simulink model "Md32StEnCtrl"  (R2018b)
settings: Solver=FixedStepDiscrete  StartTime=0.0  StopTime=10.0  FixedStep=0.01  RelTol=1e-3
undefined symbols (not defined in the file or in its folder): data, SecRwLtStBkReclnEn_Clear, SecRwLtStBkReclnEn_Set, SecRwRtStBkReclnEn_Clear, SecRwRtStBkReclnEn_Set, ThdRwLtStBkReclnEn_Clear, ThdRwLtStBkReclnEn_Set, ThdRwLtStCshnFldEn_Clear, ThdRwLtStCshnFldEn_Set
libraries: simulink x1
settings Model: Creator=sn2xws  LastModifiedBy=sn2xws
settings Model: ModifiedHistory=|
  | 2024.6.24 V3.0.0 557模式流程V1.9
  | 2024.8.16 V3.0.1函数增加FirstTrig
  | 2024.8.20 V3.0.2FirstTrig 折叠刀位置时，不再调用电机
  | 2024.12.17 V3.0.3 BUG 962485 3L靠背和2L靠背应同时进行
settings DataIOCC: SaveFormat=StructureWithTime
settings OptimizationCC: DefaultParameterBehavior=Inlined  EnhancedBackFolding=on  PassReuseOutputArgsAs=Individual arguments  ZeroExternalMemoryAtStartup=off  ZeroInternalMemoryAtStartup=off  OptimizeBlockOrder=speed  DifferentSizesBufferReuse=on  OptimizationCustomize=off
settings DebuggingCC: ParameterTunabilityLossMsg=error
settings SFSimCC: MATLABDynamicMemAlloc=off
settings RTWCC: SystemTargetFile=autosar.tlc  GenCodeOnly=on  TemplateMakefile=ert_default_tmf  Description=AUTOSAR  GenerateReport=on  IncludeHyperlinkInReport=on  LaunchReport=on  GenerateTraceInfo=on  GenerateTraceReport=on  GenerateTraceReportSl=on  GenerateTraceReportSf=on  GenerateTraceReportEml=on
settings CodeAppCC: ForceParamTrailComments=on  IgnoreCustomStorageClasses=off  OperatorAnnotations=on  SimulinkDataObjDesc=on  SFDataObjDesc=on  InsertBlockDesc=on
settings STFCustomTargetCC: TargetLangStandard=C99 (ISO)  MultiwordLength=256  ParMdlRefBuildCompliant=on  CompOptLevelCompliant=on  IncludeMdlTerminateFcn=off  CombineOutputUpdateFcns=on  SuppressErrorStatus=on  ERTCustomFileBanners=on  SupportNonFinite=off  SupportComplex=off  SupportContinuousTime=off  SupportNonInlinedSFcns=off  RemoveResetFunc=on  MATLABClassNameForMDSCustomization=Simulink.SoftwareTarget.ERTCustomization  AutosarCompliant=on  UseToolchainInfoCompliant=on  LookupTableObjectStructAxisOrder=2,1,3,4,...  LUTObjectStructOrderEvenSpacing=Size,Table,Breakpoints  SystemTargetFile=autosar.tlc
settings ERTTargetCC: TargetLangStandard=C99 (ISO)  ConcurrentExecutionCompliant=off  IncludeMdlTerminateFcn=off  SuppressErrorStatus=on  SupportNonFinite=off  SupportComplex=off  ModelStepFunctionPrototypeControlCompliant=off  CPPClassGenCompliant=off  AutosarCompliant=on  LookupTableObjectStructAxisOrder=2,1,3,4,...  LUTObjectStructOrderEvenSpacing=Size,Table,Breakpoints  InlinedParameterPlacement=NonHierarchical  ERTCustomFileTemplate=example_file_process.tlc  ERTFilePackagingFormat=Compact

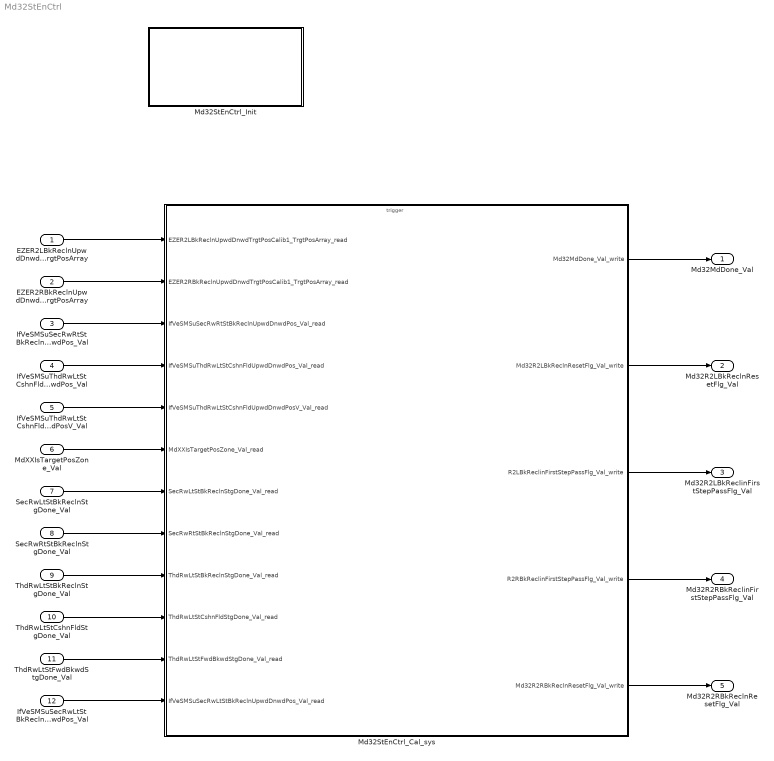
== system Md32StEnCtrl ==
  EZER2LBkReclnUpwdDnwdTrgtPosCalib1_TrgtPosArray : Inport  Description=|  OutDataTypeStr=uint16  PortDimensions=3
      | 0:Pos
      | 1:Max
      | 2:Min
  EZER2RBkReclnUpwdDnwdTrgtPosCalib1_TrgtPosArray : Inport  Description=|  Port=2  OutDataTypeStr=uint16  PortDimensions=3
      | 0:Pos
      | 1:Max
      | 2:Min
  IfVeSMSuSecRwRtStBkReclnUpwdDnwdPos_Val : Inport  Port=3  OutDataTypeStr=uint16  PortDimensions=1
  IfVeSMSuThdRwLtStCshnFldUpwdDnwdPos_Val : Inport  Port=4  OutDataTypeStr=uint16  PortDimensions=1
  IfVeSMSuThdRwLtStCshnFldUpwdDnwdPosV_Val : Inport  Port=5  OutDataTypeStr=boolean  PortDimensions=1
  MdXXIsTargetPosZone_Val : Inport  Port=6  OutDataTypeStr=uint32  PortDimensions=1
  SecRwLtStBkReclnStgDone_Val : Inport  Port=7  OutDataTypeStr=boolean  PortDimensions=1
  SecRwRtStBkReclnStgDone_Val : Inport  Port=8  OutDataTypeStr=boolean  PortDimensions=1
  ThdRwLtStBkReclnStgDone_Val : Inport  Port=9  OutDataTypeStr=boolean  PortDimensions=1
  ThdRwLtStCshnFldStgDone_Val : Inport  Port=10  OutDataTypeStr=boolean  PortDimensions=1
  ThdRwLtStFwdBkwdStgDone_Val : Inport  Port=11  OutDataTypeStr=boolean  PortDimensions=1
  IfVeSMSuSecRwLtStBkReclnUpwdDnwdPos_Val : Inport  Port=12  OutDataTypeStr=uint16  PortDimensions=1
  Md32StEnCtrl_Cal_sys : Subsystem
  Md32StEnCtrl_Init : Subsystem
  Md32MdDone_Val : Outport  OutDataTypeStr=uint8  PortDimensions=1
  Md32R2LBkReclnResetFlg_Val : Outport  Port=2  OutDataTypeStr=boolean  PortDimensions=1
  Md32R2LBkReclinFirstStepPassFlg_Val : Outport  Port=3  OutDataTypeStr=boolean  PortDimensions=1
  Md32R2RBkReclinFirstStepPassFlg_Val : Outport  Port=4  OutDataTypeStr=boolean  PortDimensions=1
  Md32R2RBkReclnResetFlg_Val : Outport  Port=5  OutDataTypeStr=boolean  PortDimensions=1
  wires:
  EZER2LBkReclnUpwdDnwdTrgtPosCalib1_TrgtPosArray/1 -> Md32StEnCtrl_Cal_sys/1(EZER2LBkReclnUpwdDnwdTrgtPosCalib1_TrgtPosArray_read)
  EZER2RBkReclnUpwdDnwdTrgtPosCalib1_TrgtPosArray/1 -> Md32StEnCtrl_Cal_sys/2(EZER2RBkReclnUpwdDnwdTrgtPosCalib1_TrgtPosArray_read)
  IfVeSMSuSecRwRtStBkReclnUpwdDnwdPos_Val/1 -> Md32StEnCtrl_Cal_sys/3(IfVeSMSuSecRwRtStBkReclnUpwdDnwdPos_Val_read)
  IfVeSMSuThdRwLtStCshnFldUpwdDnwdPos_Val/1 -> Md32StEnCtrl_Cal_sys/4(IfVeSMSuThdRwLtStCshnFldUpwdDnwdPos_Val_read)
  IfVeSMSuThdRwLtStCshnFldUpwdDnwdPosV_Val/1 -> Md32StEnCtrl_Cal_sys/5(IfVeSMSuThdRwLtStCshnFldUpwdDnwdPosV_Val_read)
  MdXXIsTargetPosZone_Val/1 -> Md32StEnCtrl_Cal_sys/6(MdXXIsTargetPosZone_Val_read)
  SecRwLtStBkReclnStgDone_Val/1 -> Md32StEnCtrl_Cal_sys/7(SecRwLtStBkReclnStgDone_Val_read)
  SecRwRtStBkReclnStgDone_Val/1 -> Md32StEnCtrl_Cal_sys/8(SecRwRtStBkReclnStgDone_Val_read)
  ThdRwLtStBkReclnStgDone_Val/1 -> Md32StEnCtrl_Cal_sys/9(ThdRwLtStBkReclnStgDone_Val_read)
  ThdRwLtStCshnFldStgDone_Val/1 -> Md32StEnCtrl_Cal_sys/10(ThdRwLtStCshnFldStgDone_Val_read)
  ThdRwLtStFwdBkwdStgDone_Val/1 -> Md32StEnCtrl_Cal_sys/11(ThdRwLtStFwdBkwdStgDone_Val_read)
  Md32StEnCtrl_Cal_sys/1(Md32MdDone_Val_write) -> Md32MdDone_Val/1
  Md32StEnCtrl_Cal_sys/2(Md32R2LBkReclnResetFlg_Val_write) -> Md32R2LBkReclnResetFlg_Val/1
  Md32StEnCtrl_Cal_sys/3(R2LBkReclinFirstStepPassFlg_Val_write) -> Md32R2LBkReclinFirstStepPassFlg_Val/1
  Md32StEnCtrl_Cal_sys/4(R2RBkReclinFirstStepPassFlg_Val_write) -> Md32R2RBkReclinFirstStepPassFlg_Val/1
  IfVeSMSuSecRwLtStBkReclnUpwdDnwdPos_Val/1 -> Md32StEnCtrl_Cal_sys/12(IfVeSMSuSecRwLtStBkReclnUpwdDnwdPos_Val_read)
  Md32StEnCtrl_Cal_sys/5(Md32R2RBkReclnResetFlg_Val_write) -> Md32R2RBkReclnResetFlg_Val/1

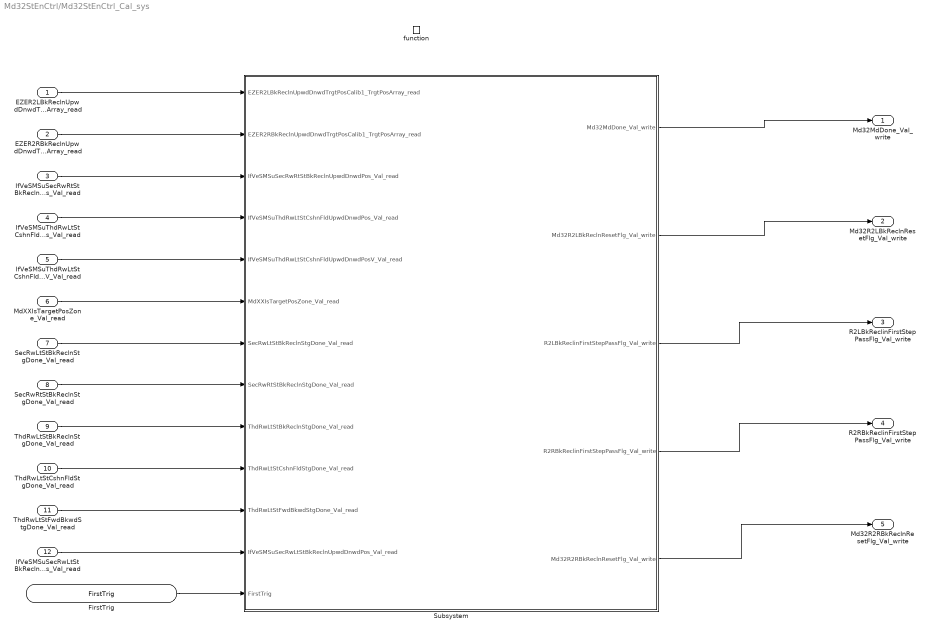
== system Md32StEnCtrl/Md32StEnCtrl_Cal_sys ==
  EZER2LBkReclnUpwdDnwdTrgtPosCalib1_TrgtPosArray_read : Inport
  EZER2RBkReclnUpwdDnwdTrgtPosCalib1_TrgtPosArray_read : Inport  Port=2
  IfVeSMSuSecRwRtStBkReclnUpwdDnwdPos_Val_read : Inport  Port=3
  IfVeSMSuThdRwLtStCshnFldUpwdDnwdPos_Val_read : Inport  Port=4
  IfVeSMSuThdRwLtStCshnFldUpwdDnwdPosV_Val_read : Inport  Port=5
  MdXXIsTargetPosZone_Val_read : Inport  Port=6
  SecRwLtStBkReclnStgDone_Val_read : Inport  Port=7
  SecRwRtStBkReclnStgDone_Val_read : Inport  Port=8
  ThdRwLtStBkReclnStgDone_Val_read : Inport  Port=9
  ThdRwLtStCshnFldStgDone_Val_read : Inport  Port=10
  ThdRwLtStFwdBkwdStgDone_Val_read : Inport  Port=11
  IfVeSMSuSecRwLtStBkReclnUpwdDnwdPos_Val_read : Inport  Port=12
  function : TriggerPort  TriggerType=function-call  IsSimulinkFunction=on  FunctionName=Md32StEnCtrl_Cal  VariantControl=(inherit)
  Subsystem : Subsystem
  FirstTrig : ArgIn  OutDataTypeStr=boolean  ArgumentName=FirstTrig
  Md32MdDone_Val_write : Outport
      settings: EnsureOutportIsVirtual=on
  Md32R2LBkReclnResetFlg_Val_write : Outport  Port=2
      settings: EnsureOutportIsVirtual=on
  R2LBkReclinFirstStepPassFlg_Val_write : Outport  Port=3
      settings: EnsureOutportIsVirtual=on
  R2RBkReclinFirstStepPassFlg_Val_write : Outport  Port=4
      settings: EnsureOutportIsVirtual=on
  Md32R2RBkReclnResetFlg_Val_write : Outport  Port=5
      settings: EnsureOutportIsVirtual=on
  wires:
  EZER2LBkReclnUpwdDnwdTrgtPosCalib1_TrgtPosArray_read/1 -> Subsystem/1(EZER2LBkReclnUpwdDnwdTrgtPosCalib1_TrgtPosArray_read)
  EZER2RBkReclnUpwdDnwdTrgtPosCalib1_TrgtPosArray_read/1 -> Subsystem/2(EZER2RBkReclnUpwdDnwdTrgtPosCalib1_TrgtPosArray_read)
  IfVeSMSuSecRwRtStBkReclnUpwdDnwdPos_Val_read/1 -> Subsystem/3(IfVeSMSuSecRwRtStBkReclnUpwdDnwdPos_Val_read)
  IfVeSMSuThdRwLtStCshnFldUpwdDnwdPos_Val_read/1 -> Subsystem/4(IfVeSMSuThdRwLtStCshnFldUpwdDnwdPos_Val_read)
  IfVeSMSuThdRwLtStCshnFldUpwdDnwdPosV_Val_read/1 -> Subsystem/5(IfVeSMSuThdRwLtStCshnFldUpwdDnwdPosV_Val_read)
  MdXXIsTargetPosZone_Val_read/1 -> Subsystem/6(MdXXIsTargetPosZone_Val_read)
  SecRwLtStBkReclnStgDone_Val_read/1 -> Subsystem/7(SecRwLtStBkReclnStgDone_Val_read)
  SecRwRtStBkReclnStgDone_Val_read/1 -> Subsystem/8(SecRwRtStBkReclnStgDone_Val_read)
  ThdRwLtStBkReclnStgDone_Val_read/1 -> Subsystem/9(ThdRwLtStBkReclnStgDone_Val_read)
  ThdRwLtStCshnFldStgDone_Val_read/1 -> Subsystem/10(ThdRwLtStCshnFldStgDone_Val_read)
  ThdRwLtStFwdBkwdStgDone_Val_read/1 -> Subsystem/11(ThdRwLtStFwdBkwdStgDone_Val_read)
  Subsystem/1(Md32MdDone_Val_write) -> Md32MdDone_Val_write/1
  Subsystem/2(Md32R2LBkReclnResetFlg_Val_write) -> Md32R2LBkReclnResetFlg_Val_write/1
  Subsystem/3(R2LBkReclinFirstStepPassFlg_Val_write) -> R2LBkReclinFirstStepPassFlg_Val_write/1
  Subsystem/4(R2RBkReclinFirstStepPassFlg_Val_write) -> R2RBkReclinFirstStepPassFlg_Val_write/1
  IfVeSMSuSecRwLtStBkReclnUpwdDnwdPos_Val_read/1 -> Subsystem/12(IfVeSMSuSecRwLtStBkReclnUpwdDnwdPos_Val_read)
  Subsystem/5(Md32R2RBkReclnResetFlg_Val_write) -> Md32R2RBkReclnResetFlg_Val_write/1
  FirstTrig/1 -> Subsystem/13(FirstTrig)

== system Md32StEnCtrl/Md32StEnCtrl_Init ==
  Event Listener : EventListener  EventName=reset

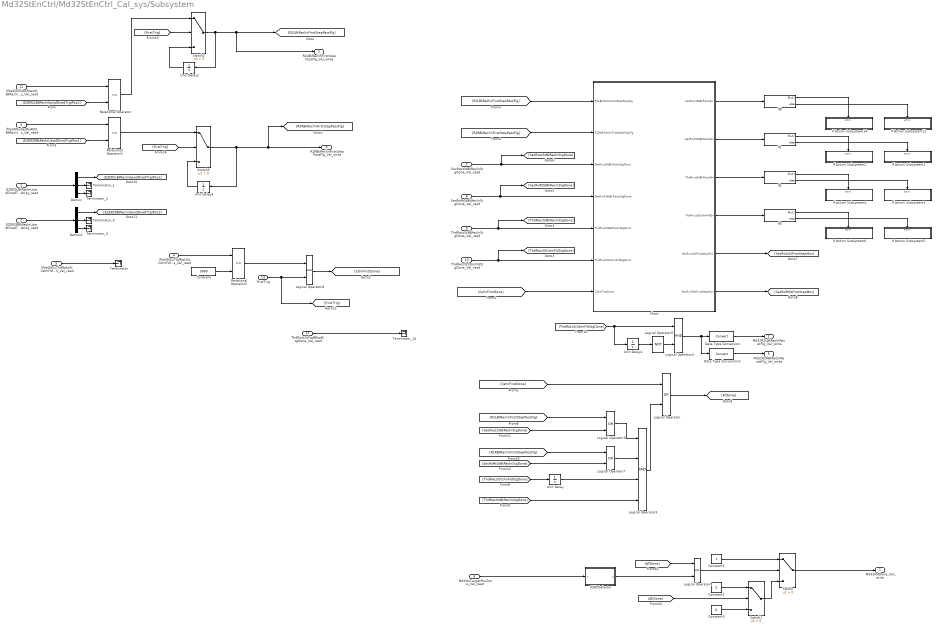
== system Md32StEnCtrl/Md32StEnCtrl_Cal_sys/Subsystem ==
  EZER2LBkReclnUpwdDnwdTrgtPosCalib1_TrgtPosArray_read : Inport
  EZER2RBkReclnUpwdDnwdTrgtPosCalib1_TrgtPosArray_read : Inport  Port=2
  IfVeSMSuSecRwRtStBkReclnUpwdDnwdPos_Val_read : Inport  Port=3
  IfVeSMSuThdRwLtStCshnFldUpwdDnwdPos_Val_read : Inport  Port=4
  IfVeSMSuThdRwLtStCshnFldUpwdDnwdPosV_Val_read : Inport  Port=5
  MdXXIsTargetPosZone_Val_read : Inport  Port=6
  SecRwLtStBkReclnStgDone_Val_read : Inport  Port=7
  SecRwRtStBkReclnStgDone_Val_read : Inport  Port=8
  ThdRwLtStBkReclnStgDone_Val_read : Inport  Port=9
  ThdRwLtStCshnFldStgDone_Val_read : Inport  Port=10
  ThdRwLtStFwdBkwdStgDone_Val_read : Inport  Port=11
  IfVeSMSuSecRwLtStBkReclnUpwdDnwdPos_Val_read : Inport  Port=12
  FirstTrig : Inport  Port=13
  32BitSelector : Subsystem  mask(32 Bit Selector){BitNum=31}
      mask prompts: BitNum "Select Bit Number"
      mask help: Allows selection of a particular bit (0-31) out of a packed word up to 32 bits long. Output will be true if the bit number selected via the mask parameter is equal to one.
      mask TypeOptions BitNum: 0 | 1 | 2 | 3 | 4 | 5 | 6 | 7 | 8 | 9 | 10 | 11 | 12 | 13 | 14 | 15 | 16 | 17 | 18 | 19 | 20 | 21 | 22 | 23 | 24 | 25 | 26 | 27 | 28 | 29 | 30 | 31
      mask Display:
      | text(0.5, 0.8,'BIT','horizontalAlignment','center')
      | text(0.5, 0.5,'SELECTOR','horizontalAlignment','center')
      | text(0.5, 0.2,['-- Bit ',char(get_param(gcb,'BitNum')),' --'],'horizontalAlignment','center')
  Chart : Stateflow chart  TreatAsAtomicUnit=on
  Constant : Constant  Value=3960  OutDataTypeStr=uint16
  Constant1 : Constant  OutDataTypeStr=uint8
  Constant2 : Constant  Value=2  OutDataTypeStr=uint8
  Constant3 : Constant  Value=0  OutDataTypeStr=uint8
  Data Type Conversion : DataTypeConversion
  Data Type Conversion1 : DataTypeConversion
  Demux : Demux  Outputs=3
  Demux1 : Demux  Outputs=3
  If Action Subsystem1 : Subsystem  TreatAsAtomicUnit=on
  If Action Subsystem11 : Subsystem  TreatAsAtomicUnit=on
  If Action Subsystem14 : Subsystem  TreatAsAtomicUnit=on
  If Action Subsystem2 : Subsystem  TreatAsAtomicUnit=on
  If Action Subsystem3 : Subsystem  TreatAsAtomicUnit=on
  If Action Subsystem4 : Subsystem  TreatAsAtomicUnit=on
  If Action Subsystem5 : Subsystem  TreatAsAtomicUnit=on
  If Action Subsystem6 : Subsystem  TreatAsAtomicUnit=on
  If{1..3,8} (4 alike) : If  IfExpression=u1
  Logical Operator : Logic  Operator=OR  AllPortsSameDT=off  OutDataTypeStr=boolean
  Logical Operator3 : Logic  Inputs=4  AllPortsSameDT=off  OutDataTypeStr=boolean
  Logical Operator4 : Logic  AllPortsSameDT=off  OutDataTypeStr=boolean
  Logical Operator5 : Logic  Operator=NOT  AllPortsSameDT=off  OutDataTypeStr=boolean
  Logical Operator6 : Logic  Operator=OR  AllPortsSameDT=off  OutDataTypeStr=boolean
  Logical Operator7 : Logic  Operator=OR  AllPortsSameDT=off  OutDataTypeStr=boolean
  Logical Operator8 : Logic  AllPortsSameDT=off  OutDataTypeStr=boolean
  Logical Operator9 : Logic  AllPortsSameDT=off  OutDataTypeStr=boolean
  Relational Operator : RelationalOperator  Operator=<=  OutDataTypeStr=boolean  RndMeth=Simplest
  Relational Operator1 : RelationalOperator  Operator=<=  OutDataTypeStr=boolean  RndMeth=Simplest
  Relational Operator2 : RelationalOperator  OutDataTypeStr=boolean  RndMeth=Simplest
  Switch{,1..3} (4 alike) : Switch  Criteria=u2 > Threshold
  Terminator : Terminator
  Terminator_{1..4,14} (5 alike) : Terminator
  Unit Delay{,1..3} (4 alike) : UnitDelay  SampleTime=-1
  Md32MdDone_Val_write : Outport
      settings: EnsureOutportIsVirtual=on
  Md32R2LBkReclnResetFlg_Val_write : Outport  Port=2
      settings: EnsureOutportIsVirtual=on
  R2LBkReclinFirstStepPassFlg_Val_write : Outport  Port=3
      settings: EnsureOutportIsVirtual=on
  R2RBkReclinFirstStepPassFlg_Val_write : Outport  Port=4
      settings: EnsureOutportIsVirtual=on
  Md32R2RBkReclnResetFlg_Val_write : Outport  Port=5
      settings: EnsureOutportIsVirtual=on
  wires:
  IfVeSMSuThdRwLtStCshnFldUpwdDnwdPos_Val_read/1 -> Relational Operator2/1
  ThdRwLtStFwdBkwdStgDone_Val_read/1 -> Terminator_14/1
  IfVeSMSuSecRwLtStBkReclnUpwdDnwdPos_Val_read/1 -> Relational Operator/1
  IfVeSMSuSecRwRtStBkReclnUpwdDnwdPos_Val_read/1 -> Relational Operator1/1
  Constant/1 -> Relational Operator2/2
  IfVeSMSuThdRwLtStCshnFldUpwdDnwdPosV_Val_read/1 -> Terminator/1
  [CshnFirstDone] -> Logical Operator/1
  [R2RBkReclinFirstStepPassFlg] -> Chart/2(R2RBkReclinFirstStepPassFlg)
  [R2LBkReclinFirstStepPassFlg] -> Chart/1(R2LBkReclinFirstStepPassFlg)
  SecRwLtStBkReclnStgDone_Val_read/1 -> [SecRwLtStBkReclnStgDone], Chart/3(SecRwLtStBkReclnStgDone)
  SecRwRtStBkReclnStgDone_Val_read/1 -> [SecRwRtStBkReclnStgDone], Chart/4(SecRwRtStBkReclnStgDone)
  ThdRwLtStBkReclnStgDone_Val_read/1 -> [ThdRwLtStBkReclnStgDone], Chart/5(ThdRwLtStBkReclnStgDone)
  ThdRwLtStCshnFldStgDone_Val_read/1 -> [ThdRwLtStCshnFldStgDone], Chart/6(ThdRwLtStCshnFldStgDone)
  [CshnFirstDone] -> Chart/7(CshnFirstDone)
  Chart/5(SecRwLtStFirstStepMov) -> [SecRwLtStFirstStepMov]
  Chart/6(SecRwRtStFirstStepMov) -> [SecRwRtStFirstStepMov]
  [ThdRwLtStBkReclnStgDone] -> Logical Operator3/4
  [ThdRwLtStCshnFldStgDone] -> Unit Delay/1
  Logical Operator3/1 -> Logical Operator/2
  Unit Delay/1 -> Logical Operator3/3
  [ThdRwLtStCshnFldStgDone] -> Unit Delay1/1, Logical Operator4/1
  Unit Delay1/1 -> Logical Operator5/1
  Logical Operator5/1 -> Logical Operator4/2
  Logical Operator4/1 -> Data Type Conversion1/1, Data Type Conversion/1
  Logical Operator/1 -> [AllDone]
  [R2LBkReclinFirstStepPassFlg] -> Logical Operator6/1
  [SecRwLtStBkReclnStgDone] -> Logical Operator6/2
  Logical Operator6/1 -> Logical Operator3/1
  Logical Operator7/1 -> Logical Operator3/2
  [R2RBkReclinFirstStepPassFlg] -> Logical Operator7/1
  [SecRwRtStBkReclnStgDone] -> Logical Operator7/2
  32BitSelector/1(y) -> Logical Operator9/2
  Constant2/1 -> Switch1/1
  Switch/1 -> Md32MdDone_Val_write/1
  MdXXIsTargetPosZone_Val_read/1 -> 32BitSelector/1(x)
  [AllDone] -> Switch1/2
  Logical Operator9/1 -> Switch/2
  Constant1/1 -> Switch/1
  Constant3/1 -> Switch1/3
  Switch1/1 -> Switch/3
  If8/2 -> If Action Subsystem11/Action
  If8/1 -> If Action Subsystem14/Action
  Chart/1(SecRwLtStBkReclnEn) -> If8/1
  Chart/2(SecRwRtStBkReclnEn) -> If1/1
  If1/1 -> If Action Subsystem2/Action
  If1/2 -> If Action Subsystem1/Action
  If2/2 -> If Action Subsystem3/Action
  If2/1 -> If Action Subsystem4/Action
  Chart/3(ThdRwLtStBkReclnEn) -> If2/1
  Chart/4(ThdRwLtStCshnFldEn) -> If3/1
  If3/1 -> If Action Subsystem6/Action
  If3/2 -> If Action Subsystem5/Action
  EZER2RBkReclnUpwdDnwdTrgtPosCalib1_TrgtPosArray_read/1 -> Demux1/1
  Demux1/2 -> Terminator_3/1
  EZER2LBkReclnUpwdDnwdTrgtPosCalib1_TrgtPosArray_read/1 -> Demux/1
  Demux1/3 -> Terminator_4/1
  Demux/1 -> [EZER2LBkReclnUpwdDnwdTrgtPos1]
  Demux/2 -> Terminator_1/1
  Demux/3 -> Terminator_2/1
  Demux1/1 -> [EZER2RBkReclnUpwdDnwdTrgtPos1]
  [EZER2LBkReclnUpwdDnwdTrgtPos1] -> Relational Operator/2
  [EZER2RBkReclnUpwdDnwdTrgtPos1] -> Relational Operator1/2
  Data Type Conversion/1 -> Md32R2LBkReclnResetFlg_Val_write/1
  Data Type Conversion1/1 -> Md32R2RBkReclnResetFlg_Val_write/1
  [AllDone] -> Logical Operator9/1
  Logical Operator8/1 -> [CshnFirstDone]
  FirstTrig/1 -> [FirstTrig], Logical Operator8/2
  Relational Operator2/1 -> Logical Operator8/1
  [FirstTrig] -> Switch2/2
  Relational Operator/1 -> Switch2/1
  Switch2/1 -> Unit Delay2/1, R2LBkReclinFirstStepPassFlg_Val_write/1, [R2LBkReclinFirstStepPassFlg]
  Unit Delay2/1 -> Switch2/3
  [FirstTrig] -> Switch3/2
  Relational Operator1/1 -> Switch3/1
  Switch3/1 -> Unit Delay3/1, [R2RBkReclinFirstStepPassFlg], R2RBkReclinFirstStepPassFlg_Val_write/1
  Unit Delay3/1 -> Switch3/3

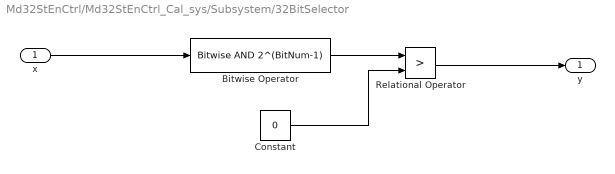
== system Md32StEnCtrl/Md32StEnCtrl_Cal_sys/Subsystem/32BitSelector ==
  x : Inport
  Bitwise Operator : simulink/Logic and Bit Operations/Bitwise Operator  logicop=AND  UseBitMask=on  BitMask=2^(BitNum-1)  BitMaskRealWorld=Stored Integer
  Constant : Constant  Value=0  OutDataTypeStr=uint32
  Relational Operator : RelationalOperator  Operator=>  OutDataTypeStr=boolean  RndMeth=Simplest
  y : Outport
  wires:
  Relational Operator/1 -> y/1
  Constant/1 -> Relational Operator/2
  x/1 -> Bitwise Operator/1
  Bitwise Operator/1 -> Relational Operator/1

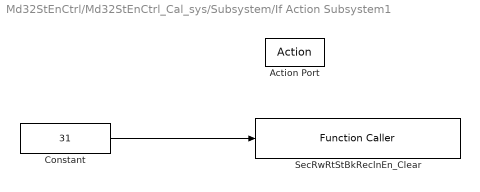
== system Md32StEnCtrl/Md32StEnCtrl_Cal_sys/Subsystem/If Action Subsystem1 ==
  Action Port : ActionPort  ActionType=else
  Constant : Constant  Value=31  OutDataTypeStr=uint8
  SecRwRtStBkReclnEn_Clear : FunctionCaller  FunctionPrototype=SecRwRtStBkReclnEn_Clear(data)  InputArgumentSpecifications=uint8(1)
  wires:
  Constant/1 -> SecRwRtStBkReclnEn_Clear/1

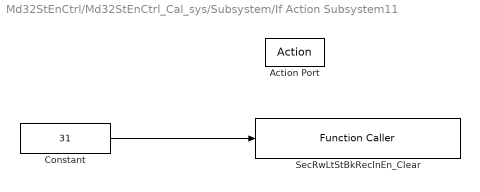
== system Md32StEnCtrl/Md32StEnCtrl_Cal_sys/Subsystem/If Action Subsystem11 ==
  Action Port : ActionPort  ActionType=else
  Constant : Constant  Value=31  OutDataTypeStr=uint8
  SecRwLtStBkReclnEn_Clear : FunctionCaller  FunctionPrototype=SecRwLtStBkReclnEn_Clear(data)  InputArgumentSpecifications=uint8(1)
  wires:
  Constant/1 -> SecRwLtStBkReclnEn_Clear/1

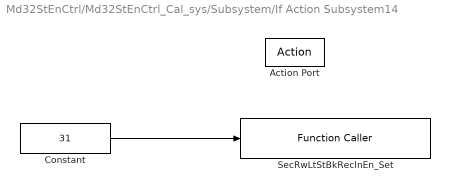
== system Md32StEnCtrl/Md32StEnCtrl_Cal_sys/Subsystem/If Action Subsystem14 ==
  Action Port : ActionPort  ActionType=then
  Constant : Constant  Value=31  OutDataTypeStr=uint8
  SecRwLtStBkReclnEn_Set : FunctionCaller  FunctionPrototype=SecRwLtStBkReclnEn_Set(data)  InputArgumentSpecifications=uint8(1)
  wires:
  Constant/1 -> SecRwLtStBkReclnEn_Set/1

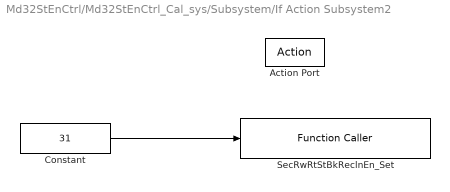
== system Md32StEnCtrl/Md32StEnCtrl_Cal_sys/Subsystem/If Action Subsystem2 ==
  Action Port : ActionPort  ActionType=then
  Constant : Constant  Value=31  OutDataTypeStr=uint8
  SecRwRtStBkReclnEn_Set : FunctionCaller  FunctionPrototype=SecRwRtStBkReclnEn_Set(data)  InputArgumentSpecifications=uint8(1)
  wires:
  Constant/1 -> SecRwRtStBkReclnEn_Set/1

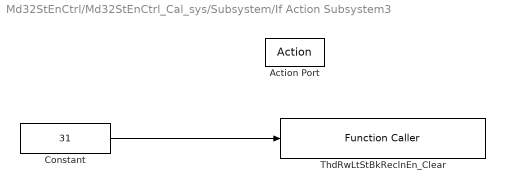
== system Md32StEnCtrl/Md32StEnCtrl_Cal_sys/Subsystem/If Action Subsystem3 ==
  Action Port : ActionPort  ActionType=else
  Constant : Constant  Value=31  OutDataTypeStr=uint8
  ThdRwLtStBkReclnEn_Clear : FunctionCaller  FunctionPrototype=ThdRwLtStBkReclnEn_Clear(data)  InputArgumentSpecifications=uint8(1)
  wires:
  Constant/1 -> ThdRwLtStBkReclnEn_Clear/1

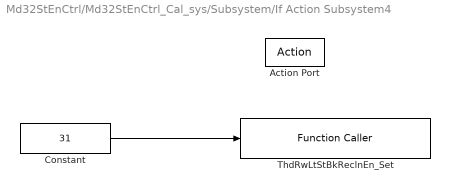
== system Md32StEnCtrl/Md32StEnCtrl_Cal_sys/Subsystem/If Action Subsystem4 ==
  Action Port : ActionPort  ActionType=then
  Constant : Constant  Value=31  OutDataTypeStr=uint8
  ThdRwLtStBkReclnEn_Set : FunctionCaller  FunctionPrototype=ThdRwLtStBkReclnEn_Set(data)  InputArgumentSpecifications=uint8(1)
  wires:
  Constant/1 -> ThdRwLtStBkReclnEn_Set/1

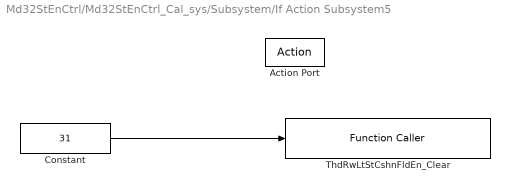
== system Md32StEnCtrl/Md32StEnCtrl_Cal_sys/Subsystem/If Action Subsystem5 ==
  Action Port : ActionPort  ActionType=else
  Constant : Constant  Value=31  OutDataTypeStr=uint8
  ThdRwLtStCshnFldEn_Clear : FunctionCaller  FunctionPrototype=ThdRwLtStCshnFldEn_Clear(data)  InputArgumentSpecifications=uint8(1)
  wires:
  Constant/1 -> ThdRwLtStCshnFldEn_Clear/1

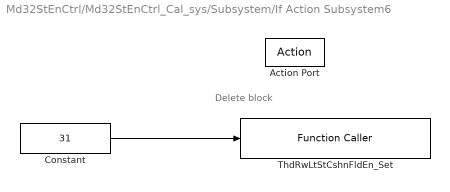
== system Md32StEnCtrl/Md32StEnCtrl_Cal_sys/Subsystem/If Action Subsystem6 ==
  note: Delete block
  Action Port : ActionPort  ActionType=then
  Constant : Constant  Value=31  OutDataTypeStr=uint8
  ThdRwLtStCshnFldEn_Set : FunctionCaller  FunctionPrototype=ThdRwLtStCshnFldEn_Set(data)  InputArgumentSpecifications=uint8(1)
  wires:
  Constant/1 -> ThdRwLtStCshnFldEn_Set/1

== stateflow chart Md32StEnCtrl/Md32StEnCtrl_Cal_sys/Subsystem/Chart ==
  (default) -> (junction 83) : {
      | SecRwLtStBkReclnEn = 0;
      | SecRwRtStBkReclnEn = 0;
      | ThdRwLtStCshnFldEn = 0;
      | ThdRwLtStBkReclnEn = 0;
      | }
  (junction 83) -> (junction 85) [order 1] : [CshnFirstDone]
  (junction 83) -> (junction 13) [order 2]
  (junction 85) -> (junction 87)
  (junction 13) -> (junction 18) [order 1] : [R2LBkReclinFirstStepPassFlg||SecRwLtStBkReclnStgDone]
  (junction 13) -> (junction 22) [order 2] : {
      | SecRwLtStBkReclnEn = 1;
      | }
  (junction 18) -> (junction 20)
  (junction 20) -> (junction 22)
  (junction 22) -> (junction 25)
  (junction 25) -> (junction 27) [order 1] : [R2RBkReclinFirstStepPassFlg ||SecRwRtStBkReclnStgDone]
  (junction 25) -> (junction 31) [order 2] : {
      | SecRwRtStBkReclnEn = 1;
      | }
  (junction 27) -> (junction 29)
  (junction 29) -> (junction 31)
  (junction 31) -> (junction 34)
  (junction 34) -> (junction 36) [order 1] : [(R2LBkReclinFirstStepPassFlg||SecRwLtStBkReclnStgDone) &&...
      | (R2RBkReclinFirstStepPassFlg ||SecRwRtStBkReclnStgDone)]
  (junction 36) -> (junction 43) [order 1] : [ThdRwLtStCshnFldStgDone]
  (junction 34) -> (junction 75) [order 2]
  (junction 36) -> (junction 38) [order 2] : {ThdRwLtStCshnFldEn = 1;}
  (junction 43) -> (junction 45)
  (junction 38) -> (junction 75)
  (junction 45) -> (junction 38)
  (junction 75) -> (junction 78)
  (junction 78) -> (junction 90) [order 1] : [ThdRwLtStCshnFldStgDone]
  (junction 90) -> (junction 100) [order 1] : [ThdRwLtStBkReclnStgDone]
  (junction 78) -> (junction 94) [order 2]
  (junction 90) -> (junction 92) [order 2] : {
      | ThdRwLtStBkReclnEn =1;
      | }
  (junction 100) -> (junction 101)
  (junction 92) -> (junction 94)
  (junction 101) -> (junction 92)
  (junction 87) -> (junction 101)
  (junction 94) -> (junction 103)
  data: R2LBkReclinFirstStepPassFlg input; R2RBkReclinFirstStepPassFlg input; SecRwLtStBkReclnStgDone input; SecRwRtStBkReclnStgDone input; ThdRwLtStBkReclnStgDone input; ThdRwLtStCshnFldStgDone input; SecRwLtStBkReclnEn output boolean; SecRwRtStBkReclnEn output boolean; ThdRwLtStBkReclnEn output boolean; ThdRwLtStCshnFldEn output boolean; CshnFirstDone input; SecRwLtStFirstStepMov output boolean; SecRwRtStFirstStepMov output boolean
